simulink model "tempcontrol_sf"  (R2022a)
settings: Solver=ode3  StartTime=0.0  StopTime=inf  FixedStep=.01  RelTol=1e-3
settings Model: ExtModeTrigDuration=2  Creator=The MathWorks, Inc.  LastModifiedBy=ndawar
settings SolverCC: AlgebraicLoopSolver=TrustRegion
settings DataIOCC: LimitDataPoints=on  SaveFormat=Array  ReturnWorkspaceOutputs=off
settings OptimizationCC: DefaultParameterBehavior=Inlined  ExpressionDepthLimit=2147483647  LifeSpan=Inf  MaxStackSize=64  EfficientTunableParamExpr=on
settings DebuggingCC: UnderspecifiedInitializationDetection=Classic  MergeDetectMultiDrivingBlocksExec=none  InheritedTsInSrcMsg=none  ParameterOverflowMsg=none  ParameterPrecisionLossMsg=none  FcnCallInpInsideContextMsg=warning  UnconnectedInputMsg=warning  UnconnectedOutputMsg=warning  UnconnectedLineMsg=warning  AllowSymbolicDim=off  StateNameClashWarn=warning  SFUnexpectedBacktrackingDiag=warning  SFNoUnconditionalDefaultTransitionDiag=warning  SFExecutionAtInitializationDiag=none  SFMachineParentedDataDiag=warning  ArithmeticOperatorsInVariantConditions=warning
settings HardwareCC: ProdBitPerInt=16  ProdBitPerPointer=16  ProdBitPerSizeT=16  ProdBitPerPtrDiffT=16  ProdLargestAtomicFloat=None  ProdWordSize=8  ProdHWDeviceType=Atmel->AVR  UseEmbeddedCoderFeatures=off  UseSimulinkCoderFeatures=off
settings ModelReferenceCC: PropagateSignalLabelsOutOfModel=off
settings SFSimCC: SimUseLocalCustomCode=off  MATLABDynamicMemAlloc=off  CustomCodeUndefinedFunction=UseInterfaceOnly
settings RTWCC: SystemTargetFile=ert.tlc  TemplateMakefile=ert_default_tmf  GenerateReport=on  RTWVerbose=off  RTWUseLocalCustomCode=off  Toolchain=Arduino AVR  BuildConfiguration=Faster Runs  LaunchReport=on
settings CodeAppCC: ForceParamTrailComments=on  OperatorAnnotations=on  MangleLength=10  StateflowObjectComments=on  MATLABSourceComments=on
settings ERTTargetCC: MultiwordLength=2048  ERTCustomFileBanners=off  SupportContinuousTime=on  SupportNonInlinedSFcns=on  RemoveResetFunc=off  ModelStepFunctionPrototypeControlCompliant=off  ERTCustomFileTemplate=example_file_process.tlc
settings ConfigComp: CovMetricSettings=dw  CovSaveCumulativeToWorkspaceVar=on  CovSaveSingleToWorkspaceVar=on  CovExternalEMLEnable=off  CovSFcnEnable=off

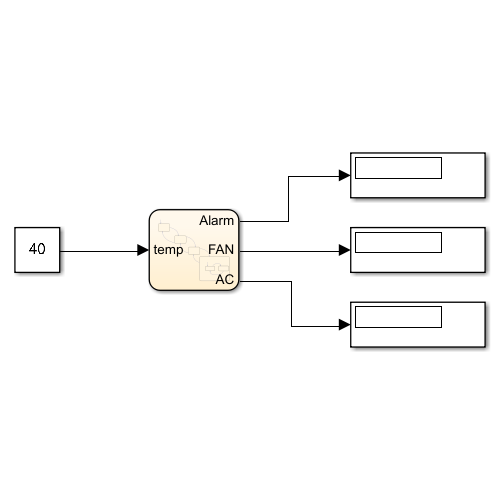
[thumbnail: Simulink's stored preview of the top-level diagram]
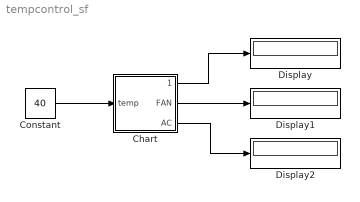
== system tempcontrol_sf ==
  Chart : Stateflow chart  TreatAsAtomicUnit=on
  Constant : Constant  Value=40  OutDataTypeStr=uint8
  Display : Display
  Display1 : Display
  Display2 : Display
  wires:
  Constant/1 -> Chart/1(temp)
  Chart/1(Alarm) -> Display/1
  Chart/2(FAN) -> Display1/1
  Chart/3(AC) -> Display2/1

== stateflow chart tempcontrol_sf/Chart ==
  state No
    FAN=false;
    AC=false;
    Alarm=false;
  state FAN_ON
    FAN=true;
    AC=false;
    Alarm=false;
  state AC_ON
    FAN=true;
    AC=true;
    Alarm=false;
  state ALARM_ON
    FAN=true;
    AC=true;
    state BlinkON
      Alarm=true;
    state BlinkOFF
      Alarm=false;
    (default) -> BlinkOFF
    BlinkOFF -> BlinkON : [after(2,sec)]
    BlinkON -> BlinkOFF : after(2,sec)
  (default) -> No
  No -> FAN_ON : [temp>70]
  FAN_ON -> No [order 1] : [temp<70]
  FAN_ON -> AC_ON [order 2] : [temp>120]
  AC_ON -> FAN_ON [order 1] : [temp<120]
  AC_ON -> ALARM_ON [order 2] : [temp>160]
  ALARM_ON -> AC_ON : [temp<160]
  data: temp input uint8; Alarm output boolean; FAN output boolean; AC output boolean
